simulink model "Controller"  (R2023a)
settings: Solver=FixedStepAuto  StartTime=0.0  StopTime=35  FixedStep=0.01  RelTol=1e-3
values from neighbouring files (symbols this model uses):
  CS_PID_psi0 = 0    [Startup_CAR_SMC.m]
  CS_PID_psid0 = 0    [Startup_CAR_SMC.m]
  CS_PID_y0 = 0    [Startup_CAR_SMC.m]
  CS_PID_yd0 = 0    [Startup_CAR_SMC.m]
undefined symbols (not defined in the file or in its folder): DiscIntNeverNeededParam
libraries: simulink x1
settings Model: Creator=Z0150218  LastModifiedBy=Z0150218

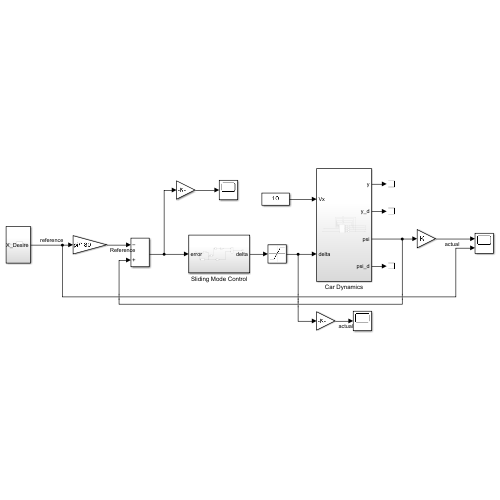
[thumbnail: Simulink's stored preview of the top-level diagram]
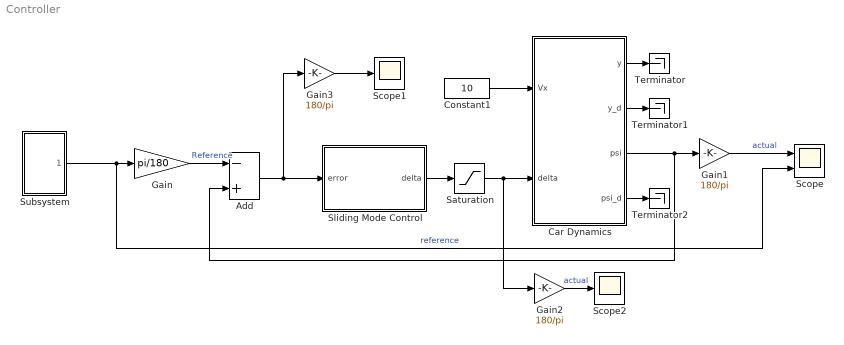
== system Controller ==
  Add : Sum  Inputs=-+
  Car Dynamics : Subsystem
  Constant1 : Constant  Value=10
  Gain : Gain  Gain=pi/180
  Gain1 : Gain  Gain=180/pi
  Gain2 : Gain  Gain=180/pi
  Gain3 : Gain  Gain=180/pi
  Saturation : Saturate  UpperLimit=deg2rad(30)  LowerLimit=-deg2rad(30)
  Scope : Scope  NumInputPorts=2
  Scope1 : Scope
  Scope2 : Scope
  Sliding Mode Control : Subsystem
  Subsystem : Subsystem
  Terminator : Terminator
  Terminator1 : Terminator
  Terminator2 : Terminator
  wires:
  Constant1/1 -> Car Dynamics/1(Vx)
  Car Dynamics/1(y) -> Terminator/1
  Car Dynamics/2(y_d) -> Terminator1/1
  Car Dynamics/3(psi) -> Add/2, Gain1/1
  Car Dynamics/4(psi_d) -> Terminator2/1
  Subsystem/1(X_Desire) -> Scope/2, Gain/1  "reference"
  Add/1 -> Gain3/1, Sliding Mode Control/1(error)
  Sliding Mode Control/1(delta) -> Saturation/1
  Gain/1 -> Add/1  "Reference"
  Saturation/1 -> Gain2/1, Car Dynamics/2(delta)
  Gain1/1 -> Scope/1  "actual"
  Gain3/1 -> Scope1/1
  Gain2/1 -> Scope2/1  "actual"

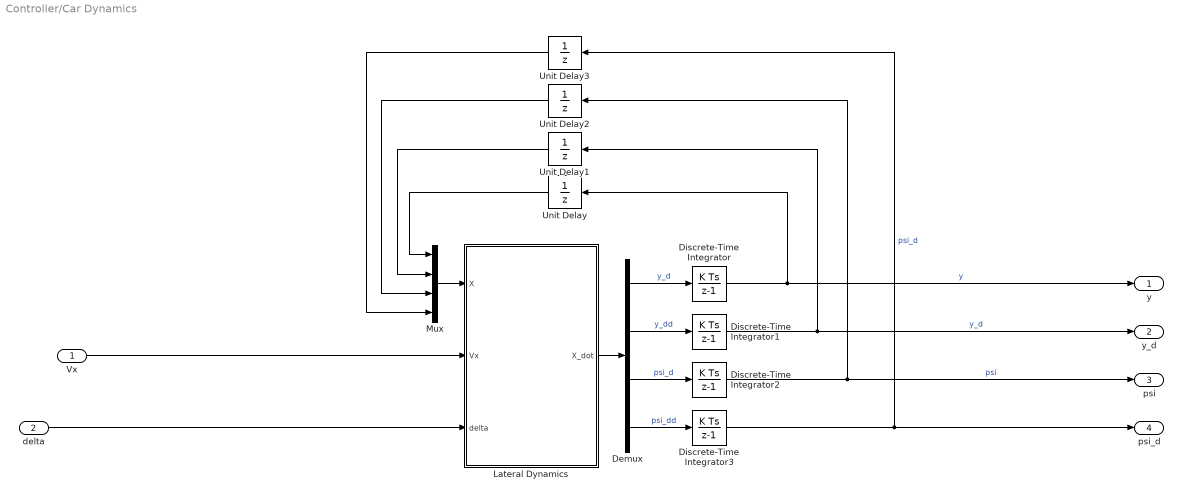
== system Controller/Car Dynamics ==
  Vx : Inport
  delta : Inport  Port=2
  Demux : Demux
  Discrete-Time Integrator{,1..3} (4 alike) : DiscreteIntegrator  SampleTime=-1  ICPrevOutput=DiscIntNeverNeededParam  ICPrevScaledInput=DiscIntNeverNeededParam
  Lateral Dynamics : MATLAB Function  TreatAsAtomicUnit=on
  Mux : Mux
  Unit Delay : UnitDelay  InitialCondition=CS_PID_y0  SampleTime=-1  HasFrameUpgradeWarning=on
  Unit Delay1 : UnitDelay  InitialCondition=CS_PID_yd0  SampleTime=-1  HasFrameUpgradeWarning=on
  Unit Delay2 : UnitDelay  InitialCondition=CS_PID_psi0  SampleTime=-1  HasFrameUpgradeWarning=on
  Unit Delay3 : UnitDelay  InitialCondition=CS_PID_psid0  SampleTime=-1  HasFrameUpgradeWarning=on
  y : Outport
  y_d : Outport  Port=2
  psi : Outport  Port=3
  psi_d : Outport  Port=4
  wires:
  Demux/1 -> Discrete-Time Integrator/1  "y_d"
  Unit Delay1/1 -> Mux/2
  Unit Delay3/1 -> Mux/4
  Discrete-Time Integrator/1 -> y/1, Unit Delay/1  "y"
  Mux/1 -> Lateral Dynamics/1(X)
  Lateral Dynamics/1(X_dot) -> Demux/1
  Discrete-Time Integrator3/1 -> psi_d/1, Unit Delay3/1  "psi_d"
  Discrete-Time Integrator1/1 -> y_d/1, Unit Delay1/1  "y_d"
  Vx/1 -> Lateral Dynamics/2(Vx)
  Unit Delay2/1 -> Mux/3
  Unit Delay/1 -> Mux/1
  Demux/3 -> Discrete-Time Integrator2/1  "psi_d"
  Demux/2 -> Discrete-Time Integrator1/1  "y_dd"
  Discrete-Time Integrator2/1 -> psi/1, Unit Delay2/1  "psi"
  Demux/4 -> Discrete-Time Integrator3/1  "psi_dd"
  delta/1 -> Lateral Dynamics/3(delta)

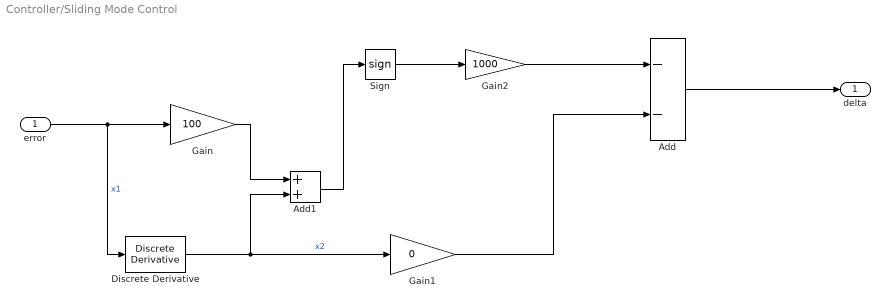
== system Controller/Sliding Mode Control ==
  error : Inport
  Add : Sum  Inputs=--
  Add1 : Sum
  Discrete Derivative : simulink/Discrete/Discrete Derivative  gainval=1.0  ICPrevScaledInput=0.0  OutMin=[]  OutMax=[]  OutDataType=fixdt(1, 16)  OutScaling=2^-10  DoSatur=off
  Gain : Gain  Gain=100
  Gain1 : Gain  Gain=0
  Gain2 : Gain  Gain=1000
  Sign : Signum
  delta : Outport
  wires:
  error/1 -> Discrete Derivative/1, Gain/1  "x1"
  Add/1 -> delta/1
  Discrete Derivative/1 -> Add1/2, Gain1/1  "x2"
  Gain/1 -> Add1/1
  Gain1/1 -> Add/2
  Add1/1 -> Sign/1
  Sign/1 -> Gain2/1
  Gain2/1 -> Add/1

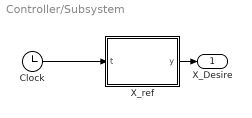
== system Controller/Subsystem ==
  Clock : Clock
  X_ref : MATLAB Function  TreatAsAtomicUnit=on
  X_Desire : Outport
  wires:
  Clock/1 -> X_ref/1(t)
  X_ref/1(y) -> X_Desire/1

== matlab function Controller/Car Dynamics/Lateral Dynamics ==
  data: X input; X_dot output; Vx input; delta input
function X_dot = fcn(X,Vx,delta)

Calpha_f = 100000;
Calpha_r = 126000;
m = 2325;
Iz = 4132;
lr = 2;
lf = 2;

A22 = -((2*Calpha_f)+(2*Calpha_r))/(m*Vx);
A24 = -Vx - ((2*Calpha_f*lf)-(2*Calpha_r*lr))/(m*Vx);
A42 = -((2*lf*Calpha_f)-(2*lr*Calpha_r))/(Iz*Vx);
A44 = -((2*(lf^2)*Calpha_f)+(2*(lr^2)*Calpha_r))/(Iz*Vx);

B21 = 2*Calpha_f/m;
B41 = (2*lf*Calpha_f)/Iz;

A = [0 1 0 0; 0 A22 0 A24; 0 0 0 1; 0 A42 0 A44];
B = [0; B21; 0; B41];

X_dot = (A*X) + (B*delta);

== matlab function Controller/Subsystem/X_ref ==
  data: t input; y output
function y = fcn(t)
if t < 10
    y = 30;
elseif t >=10 && t <20
    y = -30;
else
    y = 30*sin(t);
end
end
